simulink model "Task_1_sim"  (R2023b)
settings: Solver=VariableStepAuto  StartTime=0.0  StopTime=13  RelTol=1e-3
settings Model: Creator=nikita  LastModifiedBy=nikita

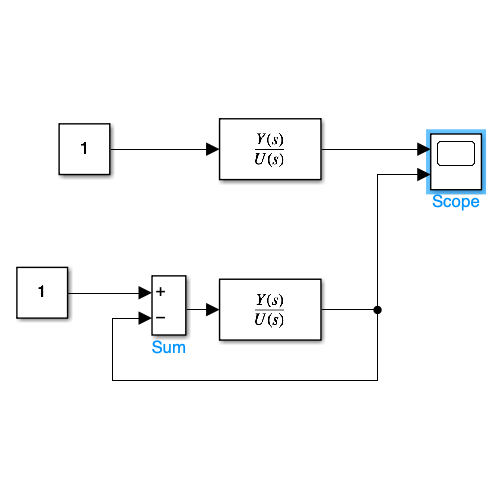
[thumbnail: Simulink's stored preview of the top-level diagram]
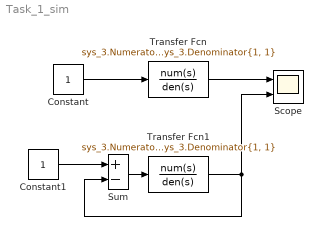
== system Task_1_sim ==
  Constant : Constant
  Constant1 : Constant
  Scope : Scope  NumInputPorts=2
  Sum : Sum  Inputs=+-
  Transfer Fcn : TransferFcn  Numerator=sys_3.Numerator{1, 1}  Denominator=sys_3.Denominator{1, 1}
  Transfer Fcn1 : TransferFcn  Numerator=sys_3.Numerator{1, 1}  Denominator=sys_3.Denominator{1, 1}
  wires:
  Constant/1 -> Transfer Fcn/1
  Transfer Fcn/1 -> Scope/1
  Sum/1 -> Transfer Fcn1/1
  Constant1/1 -> Sum/1
  Transfer Fcn1/1 -> Sum/2, Scope/2
